simulink model "test"  (Simulink 7.1)
settings: Solver=ode45  StartTime=0.0  StopTime=10.0  RelTol=1e-3
values from neighbouring files (symbols this model uses):
  ADAMS_cwd = '/home/roland/Bureau/Simulateur/SimulateurAdamsFaizRobuFASTB2'    [Controls_Plant_1.m]
  ADAMS_exec = ''    [Controls_Plant_1.m]
  ADAMS_host = 'krid.isir.upmc.fr'    [Controls_Plant_1.m]
  ADAMS_init = ''    [Controls_Plant_1.m]
  ADAMS_inputs = 'AngleBraquageAV!AngleBraquageArriere!AccelMoteur!Stab_function'    [Controls_Plant_1.m]
  ADAMS_outputs = 'PosX!PosY!PosXAvant!PosYAvant!MesureVitesse!AngleAVG!AngleAVD!AngleARG!AngleARD!VitesseRoueARD!VitesseRoueARG!VitesseLacet!roulis'    [Controls_Plant_1.m]
  ADAMS_prefix = 'Controls_Plant_1'    [Controls_Plant_1.m]
  ADAMS_static = 'yes'    [Controls_Plant_1.m]
  ADAMS_sysdir = '/home/roland/Adams/'    [Controls_Plant_1.m]
  C = ParDyn(9)    [MvtDyn.m]    (also in ParPneu.m = 1.3; Replay.m = line([X_trac(6) X_trac(8)],[Y_trac(6) Y_trac(8)],'LineWidth')
undefined symbols (not defined in the file or in its folder): Empattement, Voie
libraries: simulink x1
settings Model: Creator=roland  LastModifiedBy=roland
settings HardwareCC: ProdHWDeviceType=Generic->Unspecified (assume 32-bit Generic)

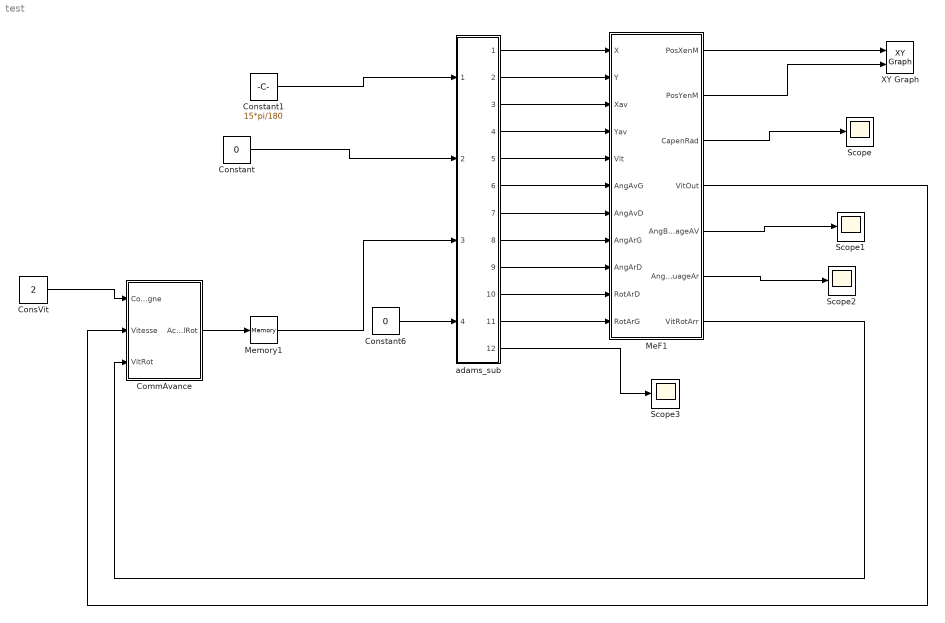
== system test ==
  CommAvance : Subsystem
  ConsVit : Constant  Value=2  OutDataType=sfix(16)  OutScaling=2^0
  Constant : Constant  Value=0  OutDataType=sfix(16)  OutScaling=2^0
  Constant1 : Constant  Value=15*pi/180  OutDataType=sfix(16)  OutScaling=2^0
  Constant6 : Constant  Value=0  OutDataType=sfix(16)  OutScaling=2^0
  MeF1 : Subsystem
  Memory1 : Memory  InheritSampleTime=on
  Scope{,1..3} (4 alike) : Scope
      Scope2 settings: SaveName=ScopeData2
      Scope3 settings: SaveName=ScopeData3
  XY Graph : simulink/Sinks/XY Graph  SystemSampleTime=-1  xmin=-1  xmax=1  ymin=-1  ymax=1  st=-1
  adams_sub : Subsystem
  wires:
  CommAvance/1(AccelRot) -> Memory1/1
  ConsVit/1 -> CommAvance/1(Consigne)
  Constant6/1 -> adams_sub/4("Stab_function       ")
  adams_sub/1("PosX          ") -> MeF1/1(X)
  adams_sub/2("PosY          ") -> MeF1/2(Y)
  adams_sub/3("PosXAvant     ") -> MeF1/3(Xav)
  adams_sub/4("PosYAvant     ") -> MeF1/4(Yav)
  adams_sub/5("AngleAVG      ") -> MeF1/5(Vit)
  adams_sub/6("AngleAVD      ") -> MeF1/6(AngAvG)
  adams_sub/7("AngleARG      ") -> MeF1/7(AngAvD)
  adams_sub/8("AngleARD      ") -> MeF1/8(AngArG)
  adams_sub/9(VitesseRoueARD) -> MeF1/9(AngArD)
  adams_sub/10(VitesseRoueARG) -> MeF1/10(RotArD)
  adams_sub/11("VitesseLacet  ") -> MeF1/11(RotArG)
  adams_sub/12("roulis        ") -> Scope3/1
  MeF1/4(VitOut) -> CommAvance/2(Vitesse)
  MeF1/7(VitRotArr) -> CommAvance/3(VitRot)
  Memory1/1 -> adams_sub/3("AccelMoteur         ")
  Constant/1 -> adams_sub/2(AngleBraquageArriere)
  Constant1/1 -> adams_sub/1("AngleBraquageAV     ")
  MeF1/1(PosXenM) -> XY Graph/1
  MeF1/2(PosYenM) -> XY Graph/2
  MeF1/3(CapenRad) -> Scope/1
  MeF1/5(AngBraquageAV) -> Scope1/1
  MeF1/6(AngBraquageAr) -> Scope2/1

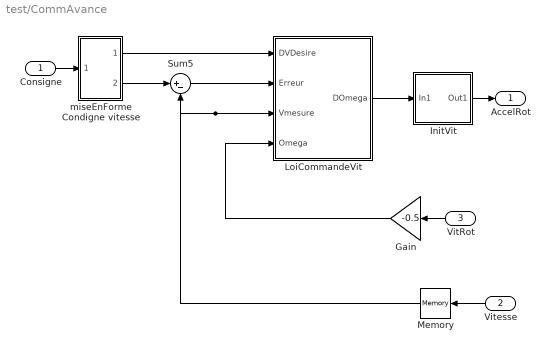
== system test/CommAvance ==
  Consigne : Inport  OutDataType=sfix(16)  OutScaling=2^0
  Vitesse : Inport  Orientation=left  Port=2  OutDataType=sfix(16)  OutScaling=2^0
  VitRot : Inport  Orientation=left  Port=3  OutDataType=sfix(16)  OutScaling=2^0
  Gain : Gain  Orientation=left  Gain=-0.5  ParameterDataType=sfix(16)  ParameterScaling=2^0  OutDataType=sfix(16)  OutScaling=2^0  SaturateOnIntegerOverflow=on  OutDataTypeStr=Inherit: Same as input  ParamDataTypeStr=Inherit: Same as input
  InitVit : Subsystem
  LoiCommandeVit : Subsystem
  Memory : Memory  Orientation=left  InheritSampleTime=on
  Sum5 : Sum  Inputs=|+-  OutDataType=sfix(16)  OutScaling=2^0  SaturateOnIntegerOverflow=on
  miseEnForme Condigne vitesse : Subsystem
  AccelRot : Outport  OutDataType=sfix(16)  OutScaling=2^0
  wires:
  LoiCommandeVit/1(DOmega) -> InitVit/1(In1)
  Sum5/1 -> LoiCommandeVit/2(Erreur)
  Gain/1 -> LoiCommandeVit/4(Omega)
  miseEnForme Condigne vitesse/2(Out2) -> Sum5/1
  miseEnForme Condigne vitesse/1(Out1) -> LoiCommandeVit/1(DVDesire)
  Memory/1 -> Sum5/2, LoiCommandeVit/3(Vmesure)
  Vitesse/1 -> Memory/1
  Consigne/1 -> miseEnForme Condigne vitesse/1(In1)
  InitVit/1(Out1) -> AccelRot/1
  VitRot/1 -> Gain/1

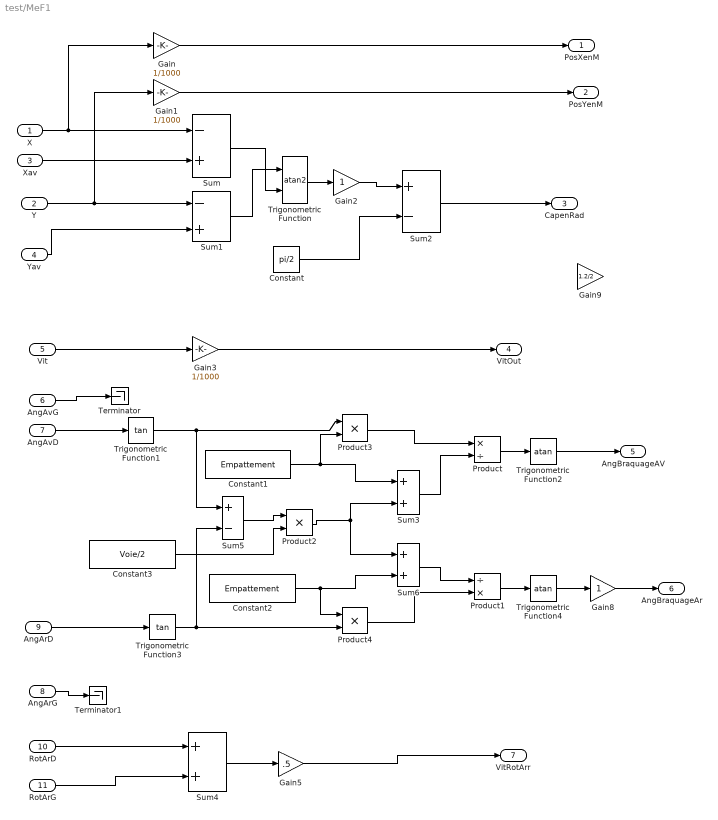
== system test/MeF1 ==
  X : Inport  OutDataType=sfix(16)  OutScaling=2^0
  Y : Inport  Port=2  OutDataType=sfix(16)  OutScaling=2^0
  Xav : Inport  Port=3  OutDataType=sfix(16)  OutScaling=2^0
  Yav : Inport  Port=4  OutDataType=sfix(16)  OutScaling=2^0
  Vit : Inport  Port=5  OutDataType=sfix(16)  OutScaling=2^0
  AngAvG : Inport  Port=6  OutDataType=sfix(16)  OutScaling=2^0
  AngAvD : Inport  Port=7  OutDataType=sfix(16)  OutScaling=2^0
  AngArG : Inport  Port=8  OutDataType=sfix(16)  OutScaling=2^0
  AngArD : Inport  Port=9  OutDataType=sfix(16)  OutScaling=2^0
  RotArD : Inport  Port=10  OutDataType=sfix(16)  OutScaling=2^0
  RotArG : Inport  Port=11  OutDataType=sfix(16)  OutScaling=2^0
  Constant : Constant  Value=pi/2  OutDataType=sfix(16)  OutScaling=2^0
  Constant1 : Constant  Value=Empattement  OutDataType=sfix(16)  OutScaling=2^0
  Constant2 : Constant  Value=Empattement  OutDataType=sfix(16)  OutScaling=2^0
  Constant3 : Constant  Value=Voie/2  OutDataType=sfix(16)  OutScaling=2^0
  Gain : Gain  Gain=1/1000  ParameterDataType=sfix(16)  ParameterScaling=2^0  OutDataType=sfix(16)  OutScaling=2^0
  Gain1 : Gain  Gain=1/1000  ParameterDataType=sfix(16)  ParameterScaling=2^0  OutDataType=sfix(16)  OutScaling=2^0
  Gain2 : Gain  ParameterDataType=sfix(16)  ParameterScaling=2^0  OutDataType=sfix(16)  OutScaling=2^0
  Gain3 : Gain  Gain=1/1000  ParameterDataType=sfix(16)  ParameterScaling=2^0  OutDataType=sfix(16)  OutScaling=2^0
  Gain5 : Gain  Gain=.5  ParameterDataType=sfix(16)  ParameterScaling=2^0  OutDataType=sfix(16)  OutScaling=2^0
  Gain8 : Gain  ParameterDataType=sfix(16)  ParameterScaling=2^0  OutDataType=sfix(16)  OutScaling=2^0
  Gain9 : Gain  Gain=1.2/2  ParameterDataType=sfix(16)  ParameterScaling=2^0  OutDataType=sfix(16)  OutScaling=2^0
  Product : Product  Inputs=*/  OutDataType=sfix(16)  OutScaling=2^0  RndMeth=Zero
  Product1 : Product  Inputs=/*  OutDataType=sfix(16)  OutScaling=2^0  RndMeth=Zero
  Product2 : Product  Inputs=**  OutDataType=sfix(16)  OutScaling=2^0  RndMeth=Zero
  Product3 : Product  Inputs=**  OutDataType=sfix(16)  OutScaling=2^0  RndMeth=Zero
  Product4 : Product  Inputs=**  OutDataType=sfix(16)  OutScaling=2^0  RndMeth=Zero
  Sum : Sum  Inputs=-+  OutDataType=sfix(16)  OutScaling=2^0
  Sum1 : Sum  Inputs=-+  OutDataType=sfix(16)  OutScaling=2^0
  Sum2 : Sum  Inputs=+-  OutDataType=sfix(16)  OutScaling=2^0
  Sum3 : Sum  OutDataType=sfix(16)  OutScaling=2^0
  Sum4 : Sum  OutDataType=sfix(16)  OutScaling=2^0
  Sum5 : Sum  Inputs=+-  OutDataType=sfix(16)  OutScaling=2^0
  Sum6 : Sum  OutDataType=sfix(16)  OutScaling=2^0
  Terminator : Terminator
  Terminator1 : Terminator
  Trigonometric Function : Trigonometry  Operator=atan2
  Trigonometric Function1 : Trigonometry  Operator=tan
  Trigonometric Function2 : Trigonometry  Operator=atan
  Trigonometric Function3 : Trigonometry  Operator=tan
  Trigonometric Function4 : Trigonometry  Operator=atan
  PosXenM : Outport  OutDataType=sfix(16)  OutScaling=2^0
  PosYenM : Outport  Port=2  OutDataType=sfix(16)  OutScaling=2^0
  CapenRad : Outport  Port=3  OutDataType=sfix(16)  OutScaling=2^0
  VitOut : Outport  Port=4  OutDataType=sfix(16)  OutScaling=2^0
  AngBraquageAV : Outport  Port=5  OutDataType=sfix(16)  OutScaling=2^0
  AngBraquageAr : Outport  Port=6  OutDataType=sfix(16)  OutScaling=2^0
  VitRotArr : Outport  Port=7  OutDataType=sfix(16)  OutScaling=2^0
  wires:
  X/1 -> Sum/1, Gain/1
  Y/1 -> Sum1/1, Gain1/1
  Xav/1 -> Sum/2
  Trigonometric Function/1 -> Gain2/1
  Yav/1 -> Sum1/2
  Gain1/1 -> PosYenM/1
  Gain2/1 -> Sum2/1
  Constant/1 -> Sum2/2
  Sum2/1 -> CapenRad/1
  Vit/1 -> Gain3/1
  Gain3/1 -> VitOut/1
  AngAvD/1 -> Trigonometric Function1/1
  Sum4/1 -> Gain5/1
  RotArD/1 -> Sum4/1
  RotArG/1 -> Sum4/2
  Gain5/1 -> VitRotArr/1
  AngArD/1 -> Trigonometric Function3/1
  AngAvG/1 -> Terminator/1
  Trigonometric Function1/1 -> Sum5/1, Product3/1
  Sum3/1 -> Product/2
  Product3/1 -> Product/1
  Product/1 -> Trigonometric Function2/1
  Trigonometric Function2/1 -> AngBraquageAV/1
  AngArG/1 -> Terminator1/1
  Trigonometric Function3/1 -> Sum5/2, Product4/2
  Constant1/1 -> Sum3/1, Product3/2
  Sum5/1 -> Product2/1
  Product2/1 -> Sum3/2, Sum6/1
  Sum6/1 -> Product1/1
  Product4/1 -> Product1/2
  Constant2/1 -> Sum6/2, Product4/1
  Product1/1 -> Trigonometric Function4/1
  Trigonometric Function4/1 -> Gain8/1
  Gain8/1 -> AngBraquageAr/1
  Sum1/1 -> Trigonometric Function/1
  Sum/1 -> Trigonometric Function/2
  Gain/1 -> PosXenM/1
  Constant3/1 -> Product2/2

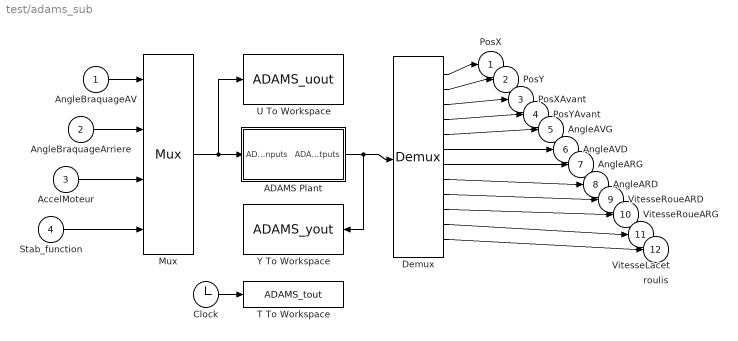
== system test/adams_sub ==
  "AngleBraquageAV     " : Inport
  AngleBraquageArriere : Inport  Port=2
  "AccelMoteur         " : Inport  Port=3
  "Stab_function       " : Inport  Port=4
  ADAMS Plant : Subsystem  mask(Adams Plant){exevie=ADAMS_sysdir, workdir=ADAMS_cwd, comtyp=PIPE(DDE), ada_host=ADAMS_host, exetyp=C++, exesol=ADAMS_exec, nampre=ADAMS_prefix, nam_in=ADAMS_inputs, namout=ADAMS_outputs, outfil=ADAMS_prefix, dt_out=0.01, o_rate=1, interorder=0, dft=no, modsim=discrete, modani=interactive, stat=ADAMS_static, inicmd=[ADAMS_init]}
      mask prompts: exevie "Adams install directory"; workdir "Adams working directory"; comtyp "Interprocess Option"; ada_host "Adams host"; exetyp "Adams solver type"; exesol "User executable (opt.: if blank - use standard)"; nampre "Adams model file prefix"; nam_in "Adams/View input names"; namout "Adams/View output names"; outfil "Output files prefix (opt.: if blank - no output)"; dt_out "Communication Interval"; o_rate "Number of communications per output step"; interorder "Interpolation Order"; dft "Direct Feedthrough"; modsim "Simulation     mode"; modani "Animation     mode"; stat "Initial Static Simulation Flag"; inicmd "Initialization commands"
      mask help: Simulate any Adams plant model either in Adams/Solver form (.adm file) or in Adams/View form (.cmd file)
      mask StyleString: edit,edit,popup(PIPE(DDE)|TCP/IP),edit,popup(Fortran|C++),edit,edit,edit,edit,edit,edit,edit,edit,popup(no|yes),popup(discrete|continuous),popup(batch|interactive),edit,edit
      mask Display: disp( 'MSCSoftware' )
  Clock : Clock
      settings: Decimation=10
  Demux : Demux  Outputs=12
  Mux : Mux
  T To Workspace : ToWorkspace  VariableName=ADAMS_tout  SaveFormat=Array
      settings: MaxDataPoints=100000
  U To Workspace : ToWorkspace  VariableName=ADAMS_uout  SaveFormat=Array
      settings: MaxDataPoints=100000
  Y To Workspace : ToWorkspace  VariableName=ADAMS_yout  SaveFormat=Array
      settings: MaxDataPoints=100000
  "PosX          " : Outport
  "PosY          " : Outport  Port=2
  "PosXAvant     " : Outport  Port=3
  "PosYAvant     " : Outport  Port=4
  "AngleAVG      " : Outport  Port=5
  "AngleAVD      " : Outport  Port=6
  "AngleARG      " : Outport  Port=7
  "AngleARD      " : Outport  Port=8
  VitesseRoueARD : Outport  Port=9
  VitesseRoueARG : Outport  Port=10
  "VitesseLacet  " : Outport  Port=11
  "roulis        " : Outport  Port=12
  wires:
  Clock/1 -> T To Workspace/1
  Mux/1 -> ADAMS Plant/1(ADAMS inputs), U To Workspace/1
  ADAMS Plant/1(ADAMS outputs) -> Demux/1, Y To Workspace/1
  Demux/1 -> "PosX          "/1
  Demux/2 -> "PosY          "/1
  Demux/3 -> "PosXAvant     "/1
  Demux/4 -> "PosYAvant     "/1
  Demux/5 -> "AngleAVG      "/1
  Demux/6 -> "AngleAVD      "/1
  Demux/7 -> "AngleARG      "/1
  Demux/8 -> "AngleARD      "/1
  Demux/9 -> VitesseRoueARD/1
  Demux/10 -> VitesseRoueARG/1
  Demux/11 -> "VitesseLacet  "/1
  Demux/12 -> "roulis        "/1
  "AngleBraquageAV     "/1 -> Mux/1
  AngleBraquageArriere/1 -> Mux/2
  "AccelMoteur         "/1 -> Mux/3
  "Stab_function       "/1 -> Mux/4

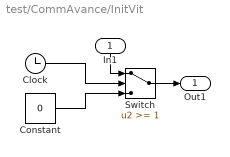
== system test/CommAvance/InitVit ==
  In1 : Inport  Orientation=down  OutDataType=sfix(16)  OutScaling=2^0
  Clock : Clock
      settings: Decimation=10
  Constant : Constant  Value=0  OutDataType=sfix(16)  OutScaling=2^0
  Switch : Switch  Threshold=1  SaturateOnIntegerOverflow=on
  Out1 : Outport  OutDataType=sfix(16)  OutScaling=2^0
  wires:
  Constant/1 -> Switch/3
  Clock/1 -> Switch/2
  In1/1 -> Switch/1
  Switch/1 -> Out1/1

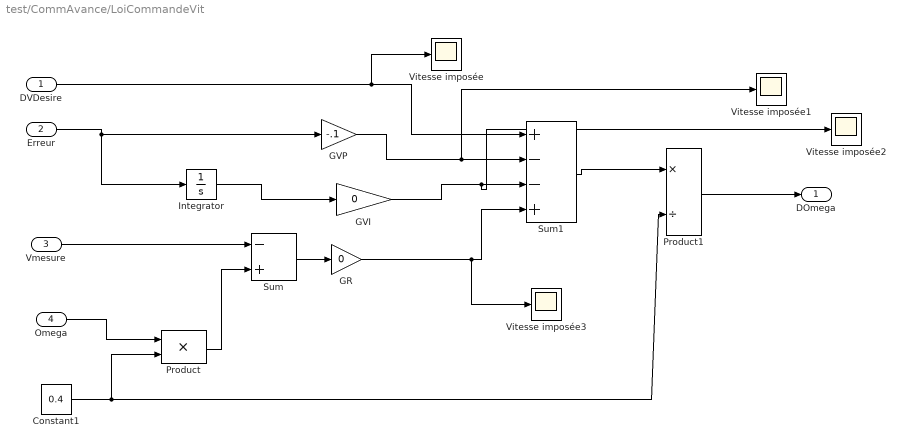
== system test/CommAvance/LoiCommandeVit ==
  DVDesire : Inport  OutDataType=sfix(16)  OutScaling=2^0
  Erreur : Inport  Port=2  OutDataType=sfix(16)  OutScaling=2^0
  Vmesure : Inport  Port=3  OutDataType=sfix(16)  OutScaling=2^0
  Omega : Inport  Port=4  OutDataType=sfix(16)  OutScaling=2^0
  Constant1 : Constant  Value=0.4  OutDataType=sfix(16)  OutScaling=2^0
  GR : Gain  Gain=0  ParameterDataType=sfix(16)  ParameterScaling=2^0  OutDataType=sfix(16)  OutScaling=2^0  SaturateOnIntegerOverflow=on  OutDataTypeStr=Inherit: Same as input  ParamDataTypeStr=Inherit: Same as input
  GVI : Gain  Gain=0  ParameterDataType=sfix(16)  ParameterScaling=2^0  OutDataType=sfix(16)  OutScaling=2^0  SaturateOnIntegerOverflow=on  OutDataTypeStr=Inherit: Same as input  ParamDataTypeStr=Inherit: Same as input
  GVP : Gain  Gain=-.1  ParameterDataType=sfix(16)  ParameterScaling=2^0  OutDataType=sfix(16)  OutScaling=2^0  SaturateOnIntegerOverflow=on  OutDataTypeStr=Inherit: Same as input  ParamDataTypeStr=Inherit: Same as input
  Integrator : Integrator
  Product : Product  OutDataType=sfix(16)  OutScaling=2^0  SaturateOnIntegerOverflow=on  OutDataTypeStr=Inherit: Same as first input
  Product1 : Product  Inputs=*/  OutDataType=sfix(16)  OutScaling=2^0  SaturateOnIntegerOverflow=on  OutDataTypeStr=Inherit: Same as first input
  Sum : Sum  Inputs=-+  OutDataType=sfix(16)  OutScaling=2^0  SaturateOnIntegerOverflow=on
  Sum1 : Sum  Inputs=+--+  OutDataType=sfix(16)  OutScaling=2^0  SaturateOnIntegerOverflow=on
  Vitesse imposée{,1..3} (4 alike) : Scope
      Vitesse imposée settings: TimeRange=12  YMin=0  YMax=2  SaveName=derivevite
      Vitesse imposée1 settings: TimeRange=12  YMin=0.0002  YMax=0.000725  SaveName=ScopeData15
      Vitesse imposée2 settings: TimeRange=12  YMin=-1  YMax=1  SaveName=ScopeData16
      Vitesse imposée3 settings: TimeRange=12  YMin=0.0425  YMax=0.0625  SaveName=ScopeData17
  DOmega : Outport  OutDataType=sfix(16)  OutScaling=2^0
  wires:
  GVI/1 -> Vitesse imposée2/1, Sum1/3
  GR/1 -> Sum1/4, Vitesse imposée3/1
  Product1/1 -> DOmega/1
  Sum1/1 -> Product1/1
  GVP/1 -> Vitesse imposée1/1, Sum1/2
  Erreur/1 -> GVP/1, Integrator/1
  DVDesire/1 -> Sum1/1, Vitesse imposée/1
  Sum/1 -> GR/1
  Vmesure/1 -> Sum/1
  Product/1 -> Sum/2
  Constant1/1 -> Product1/2, Product/2
  Omega/1 -> Product/1
  Integrator/1 -> GVI/1

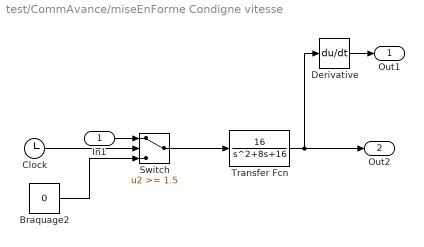
== system test/CommAvance/miseEnForme Condigne vitesse ==
  In1 : Inport  OutDataType=sfix(16)  OutScaling=2^0
  Braquage2 : Constant  Value=0  OutDataType=sfix(16)  OutScaling=2^0
  Clock : Clock
      settings: Decimation=10
  Derivative : Derivative
  Switch : Switch  Threshold=1.5
  Transfer Fcn : TransferFcn  Numerator=[16]  Denominator=[1 8 16]
  Out1 : Outport  OutDataType=sfix(16)  OutScaling=2^0
  Out2 : Outport  Port=2  OutDataType=sfix(16)  OutScaling=2^0
  wires:
  Transfer Fcn/1 -> Derivative/1, Out2/1
  Clock/1 -> Switch/2
  Braquage2/1 -> Switch/3
  Switch/1 -> Transfer Fcn/1
  Derivative/1 -> Out1/1
  In1/1 -> Switch/1

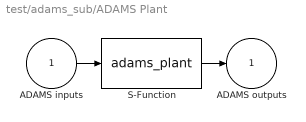
== system test/adams_sub/ADAMS Plant ==
  ADAMS inputs : Inport
  S-Function : S-Function  FunctionName=adams_plant  Parameters=exevie,exesol,stat,outfil,nampre,o_rate,nam_in,namout,dft,modsim,modani,dt_out,inicmd,exetyp,comtyp,ada_host, workdir,interorder  EnableBusSupport=off
  ADAMS outputs : Outport  InitialOutput=0
  wires:
  ADAMS inputs/1 -> S-Function/1
  S-Function/1 -> ADAMS outputs/1
